simulink model "Simulation_3DOF02"  (R2024a)
settings: Solver=ode4  StartTime=initial_time  StopTime=final_time  FixedStep=timestep  RelTol=1e-3
values from neighbouring files (symbols this model uses):
  alphaArray = [-30, -25, -20, -15, -10, -5, 0, 5, 10, 15, 20, 25, 30]    [Constants_3DOF.m]
  altitudeArray = [0, 1000, 2000, 3000, 4000, 5000, 6000, 7000, 8000, 9000, 10000, 15000, 20000,      25000, 30000, 35000, 40000, 45000, 50000, 55000, 60000]    [Constants_3DOF.m]
  cD_3DArray = zeros(numAoAs, numMachs, numAltitudes)    [Constants_3DOF.m]
  cL_3DArray = zeros(numAoAs, numMachs, numAltitudes)    [Constants_3DOF.m]
  flight_path_angle_0 = flight_path_angle_0 * (pi / 180)    (= 0.0523598775598)    [Constants_3DOF.m]
  heading_angle_0 = heading_angle_0 * (pi/180)    (= 0.349065850399)    [Constants_3DOF.m]
  height_0 = 35 * 10^3    (= 35000)    [Constants_3DOF.m]
  heightsList = usAtmosphere.Z    [Constants_3DOF.m]
  latitude_0 = latitude_0 * (pi/180)    (= 0.680503875353)    [Constants_3DOF.m]
  longitude_0 = longitude_0 * (pi/180)    (= -1.26396744429)    [Constants_3DOF.m]
  machArray = [0.5, 1.0, 1.5, 2.0, 2.5, 3.0, 3.5, 4.0, 4.5, 5.0, 5.5, 6.0, 6.5, 7.0, 7.5, 8.0,      8.5, 9.0, 9.5, 10.0]    [Constants_3DOF.m]
  mass = 161.5    [Constants_3DOF.m]
  omega_earth = 7.2921159 * 10^-5    (= 7.2921159e-05)    [Constants_3DOF.m]
  r_earth = 6371.0088 * 10^3    (= 6371008.8)    [Constants_3DOF.m]
  range_to_go_0 = 11112 * 10^3    (= 11112000)    [Constants_3DOF.m]
  rhoList = usAtmosphere.x_    [Constants_3DOF.m]
  speed_0 = 1500    [Constants_3DOF.m]
  temperatureList = usAtmosphere.T    [Constants_3DOF.m]
  wing_area = 0.079813    [Constants_3DOF.m]
libraries: simulink_extras x6
settings Model: Creator=641893  LastModifiedBy=641893

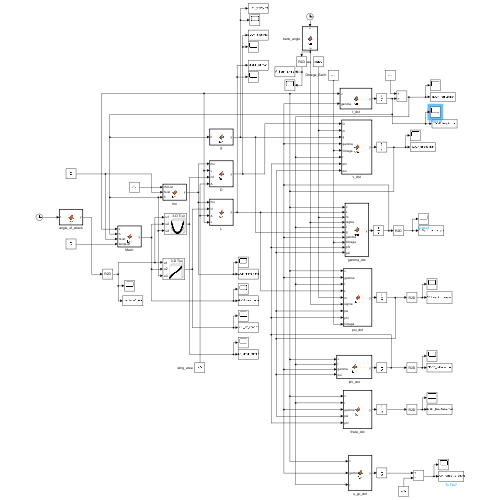
[thumbnail: Simulink's stored preview of the top-level diagram]
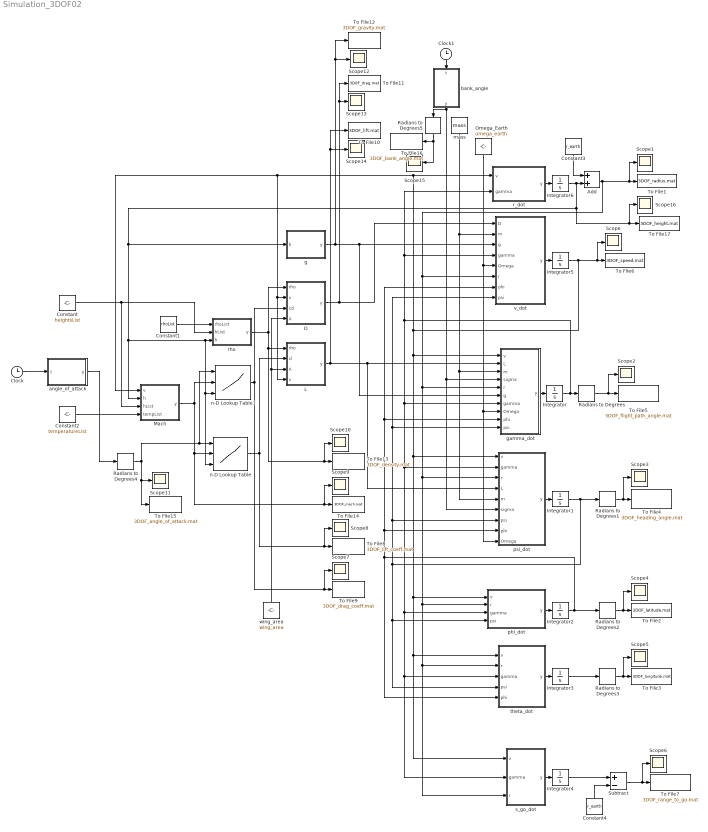
== system Simulation_3DOF02 ==
  Add : Sum
  Clock : Clock
  Clock1 : Clock
  Constant : Constant  Value=heightsList
  Constant1 : Constant  Value=rhoList
  Constant2 : Constant  Value=temperatureList
  Constant3 : Constant  Value=r_earth
  Constant4 : Constant  Value=r_earth
  D : MATLAB Function  TreatAsAtomicUnit=on
  Integrator : Integrator  InitialCondition=flight_path_angle_0
  Integrator1 : Integrator  InitialCondition=heading_angle_0
  Integrator2 : Integrator  InitialCondition=latitude_0
  Integrator3 : Integrator  InitialCondition=longitude_0
  Integrator4 : Integrator  InitialCondition=range_to_go_0
  Integrator5 : Integrator  InitialCondition=speed_0
  Integrator6 : Integrator  InitialCondition=height_0
  L : MATLAB Function  TreatAsAtomicUnit=on
  Mach : MATLAB Function  TreatAsAtomicUnit=on
  Omega_Earth : Constant  Value=omega_earth
  Radians to Degrees{,1..5} (6 alike) : simulink_extras/Transformations/Radians to Degrees
  Scope{,1..16} (17 alike) : Scope
  Subtract : Sum  Inputs=+-
  To File1 : ToFile  Filename=3DOF_radius.mat
  To File10 : ToFile  Filename=3DOF_lift.mat
  To File11 : ToFile  Filename=3DOF_drag.mat
  To File12 : ToFile  Filename=3DOF_gravity.mat
  To File13 : ToFile  Filename=3DOF_density.mat
  To File14 : ToFile  Filename=3DOF_mach.mat
  To File15 : ToFile  Filename=3DOF_angle_of_attack.mat
  To File16 : ToFile  Filename=3DOF_bank_angle.mat
  To File17 : ToFile  Filename=3DOF_height.mat
  To File2 : ToFile  Filename=3DOF_latitude.mat
  To File3 : ToFile  Filename=3DOF_longitude.mat
  To File4 : ToFile  Filename=3DOF_heading_angle.mat
  To File5 : ToFile  Filename=3DOF_flight_path_angle.mat
  To File6 : ToFile  Filename=3DOF_speed.mat
  To File7 : ToFile  Filename=3DOF_range_to_go.mat
  To File8 : ToFile  Filename=3DOF_lift_coeff.mat
  To File9 : ToFile  Filename=3DOF_drag_coeff.mat
  angle_of_attack : MATLAB Function  TreatAsAtomicUnit=on
  bank_angle : MATLAB Function  TreatAsAtomicUnit=on
  g : MATLAB Function  TreatAsAtomicUnit=on
  gamma_dot : MATLAB Function  TreatAsAtomicUnit=on
  mass : Constant  Value=mass
  n-D Lookup Table : Lookup_n-D  NumberOfTableDimensions=3  BreakpointsForDimension1=alphaArray  BreakpointsForDimension2=machArray  BreakpointsForDimension3=altitudeArray  IndexSearchMethod=Linear search  Table=cL_3DArray  InterpMethod=Linear Lagrange  InternalRulePriority=Speed  RndMeth=Simplest
      settings: InputPortMap=u0,u1,u2
  n-D Lookup Table1 : Lookup_n-D  NumberOfTableDimensions=3  BreakpointsForDimension1=alphaArray  BreakpointsForDimension2=machArray  BreakpointsForDimension3=altitudeArray  IndexSearchMethod=Linear search  Table=cD_3DArray  InterpMethod=Linear Lagrange  InternalRulePriority=Speed  RndMeth=Simplest
      settings: InputPortMap=u0,u1,u2
  phi_dot : MATLAB Function  TreatAsAtomicUnit=on
  psi_dot : MATLAB Function  TreatAsAtomicUnit=on
  r_dot : MATLAB Function  TreatAsAtomicUnit=on
  rho : MATLAB Function  TreatAsAtomicUnit=on
  s_go_dot : MATLAB Function  TreatAsAtomicUnit=on
  theta_dot : MATLAB Function  TreatAsAtomicUnit=on
  v_dot : MATLAB Function  TreatAsAtomicUnit=on
  wing_area : Constant  Value=wing_area
  wires:
  s_go_dot/1(y) -> Integrator4/1
  theta_dot/1(y) -> Integrator3/1
  phi_dot/1(y) -> Integrator2/1
  psi_dot/1(y) -> Integrator1/1
  gamma_dot/1(y) -> Integrator/1
  v_dot/1(y) -> Integrator5/1
  r_dot/1(y) -> Integrator6/1
  Integrator6/1 -> To File17/1, Scope16/1, Mach/2(h), n-D Lookup Table1/3, n-D Lookup Table/3, rho/3(h), g/1(h), Add/2
  Integrator5/1 -> Scope/1, To File6/1, L/4(v), D/2(v), Mach/1(v), r_dot/1(v), gamma_dot/1(v), psi_dot/1(v), phi_dot/1(v), theta_dot/1(v), s_go_dot/1(v)
  Integrator/1 -> r_dot/2(gamma), v_dot/4(gamma), gamma_dot/7(gamma), psi_dot/2(gamma), phi_dot/3(gamma), theta_dot/3(gamma), s_go_dot/2(gamma), Radians to Degrees/1
  Integrator1/1 -> Radians to Degrees1/1, phi_dot/4(psi), theta_dot/4(psi), psi_dot/7(psi), gamma_dot/10(psi), v_dot/8(psi)
  Integrator2/1 -> Radians to Degrees2/1, theta_dot/5(phi), psi_dot/8(phi), gamma_dot/9(phi), v_dot/7(phi)
  L/1(y) -> gamma_dot/2(L), psi_dot/4(L), Scope14/1, To File10/1
  D/1(y) -> v_dot/1(D), To File11/1, Scope13/1
  g/1(y) -> gamma_dot/6(g), v_dot/3(g), To File12/1, Scope12/1
  rho/1(y) -> L/1(rho), Scope10/1, To File13/1, D/1(rho)
  bank_angle/1(y) -> Radians to Degrees5/1, gamma_dot/4(sigma), psi_dot/6(sigma)
  angle_of_attack/1(y) -> Radians to Degrees4/1
  Clock/1 -> angle_of_attack/1(t)
  Clock1/1 -> bank_angle/1(t)
  Constant1/1 -> rho/1(rhoList)
  Constant/1 -> rho/2(hList), Mach/3(hList)
  Constant2/1 -> Mach/4(tempList)
  wing_area/1 -> L/3(A), D/4(A)
  mass/1 -> v_dot/2(m), gamma_dot/3(m), psi_dot/5(m)
  Omega_Earth/1 -> v_dot/5(Omega), gamma_dot/8(Omega), psi_dot/9(Omega)
  Add/1 -> v_dot/6(r), gamma_dot/5(r), psi_dot/3(r), phi_dot/2(r), theta_dot/2(r), s_go_dot/3(r), Scope1/1, To File1/1
  Constant3/1 -> Add/1
  Radians to Degrees/1 -> Scope2/1, To File5/1
  Radians to Degrees1/1 -> Scope3/1, To File4/1
  Radians to Degrees2/1 -> Scope4/1, To File2/1
  Integrator3/1 -> Radians to Degrees3/1
  Radians to Degrees3/1 -> Scope5/1, To File3/1
  Radians to Degrees4/1 -> n-D Lookup Table/1, n-D Lookup Table1/1, Scope11/1, To File15/1
  Radians to Degrees5/1 -> Scope15/1, To File16/1
  Mach/1(y) -> n-D Lookup Table1/2, n-D Lookup Table/2, Scope9/1, To File14/1
  n-D Lookup Table/1 -> Scope8/1, To File8/1, L/2(cl)
  n-D Lookup Table1/1 -> Scope7/1, To File9/1, D/3(cd)
  Integrator4/1 -> Subtract/1
  Subtract/1 -> Scope6/1, To File7/1
  Constant4/1 -> Subtract/2

== matlab function Simulation_3DOF02/D ==
  data: rho input; y output; v input; cd input; A input
function y = fcn(rho, v, cd, A)

y = 0.5 * rho * v^2 * A * cd;

== matlab function Simulation_3DOF02/g ==
  data: y output; h input
function y = fcn(h)
mu_earth = 3.96272 * 10^14;
rE = 6378140;
y = mu_earth / (rE + h)^2;

== matlab function Simulation_3DOF02/rho ==
  data: rhoList input; hList input; h input; y output
function y = fcn(rhoList, hList,h)

h = h / 10^3;

if h >= 0
    density = interp1(hList, rhoList, h);
else
    density = 0;
end


y = density;

== matlab function Simulation_3DOF02/angle_of_attack ==
  data: t input; y output
function y = fcn(t)

alpha = 10;
alpha = alpha * pi / 180;

y = alpha;

== matlab function Simulation_3DOF02/Mach ==
  data: v input; y output; h input; hList input; tempList input
function y = fcn(v, h, hList, tempList)

gamma = 1.4;
R = 287.05;

h = h / 10^3;

if h >= 0
    temp = interp1(hList, tempList, h);
    a = sqrt(gamma * R * temp);
    y = v/a;
else
    temp = 0;
    y = 0;
end

== matlab function Simulation_3DOF02/bank_angle ==
  data: t input; y output
function y = fcn(t)

sigma = 0;
sigma = sigma * pi / 180;

y = sigma;

== matlab function Simulation_3DOF02/phi_dot ==
  data: v input; y output; r input; gamma input; psi input
function y = fcn(v, r, gamma, psi)

y = (v / r) * cos(gamma) * sin(psi);

== matlab function Simulation_3DOF02/r_dot ==
  data: v input; y output; gamma input
function y = fcn(v, gamma)

y = v * sin(gamma);

== matlab function Simulation_3DOF02/theta_dot ==
  data: v input; y output; r input; gamma input; psi input; phi input
function y = fcn(v, r, gamma, psi, phi)

y = (v * cos(gamma) * cos(psi) ) / (r * cos(phi) );

== matlab function Simulation_3DOF02/v_dot ==
  data: D input; y output; m input; g input; gamma input; Omega input; r input; phi input; psi input
function y = fcn(D, m, g, gamma, Omega, r, phi, psi)

y = -(D / m) - g * sin(gamma) + Omega^2 * r * cos(phi) * ( sin(gamma) * cos(phi) - cos(gamma) * sin(phi) * cos(psi) );

== matlab function Simulation_3DOF02/gamma_dot ==
  data: v input; y output; L input; m input; sigma input; r input; g input; gamma input; Omega input; phi input; psi input
function y = fcn(v, L, m, sigma, r, g, gamma, Omega, phi, psi)

y = (1/v) * ( (L / m) * cos(sigma) + (( v^2 / r) - g) * cos(gamma) + 2 * Omega * v * cos(phi) * sin(psi) + Omega^2 * r * cos(phi) * ( cos(gamma) * cos(phi) - sin(gamma) * sin(phi) * cos(psi) ) );

== matlab function Simulation_3DOF02/psi_dot ==
  data: v input; y output; gamma input; r input; L input; m input; sigma input; psi input; phi input; Omega input
function y = fcn(v, gamma, r, L, m, sigma, psi, phi, Omega)

y = (1 / v) * ( (L / (m * cos(gamma))) * sin(sigma) + (v^2 /  r) * cos(gamma) * sin(psi) * tan(phi) - 2 * Omega * v * (tan(gamma) * cos(psi) * cos(phi) - sin(phi) ) + (Omega^2 * r / cos(gamma)) * sin(psi) * sin(phi) * cos(phi) );

== matlab function Simulation_3DOF02/s_go_dot ==
  data: v input; y output; gamma input; r input
function y = fcn(v, gamma, r)
rE = 6378140;
y = -v * cos(gamma) * rE / r;

== matlab function Simulation_3DOF02/L ==
  data: rho input; y output; cl input; A input; v input
function y = fcn(rho, cl, A, v)

y = 0.5 * rho * v^2 * A * cl;
